simulink model "DDS_LUT_Stream_Ex1"  (R2024a)
settings: Solver=VariableStepAuto  StartTime=0.0  StopTime=0.001  RelTol=1e-3
undefined symbols (not defined in the file): i, None, S, vsva1596, xcvc1502
libraries: aieUtilities x2, hdlUtilities x1, aieDSP x1, dspsigops x1, vmcUtilities x1
settings Model: Creator=sdegala  LastModifiedBy=robg
settings ModelReferenceCC: EnableRefExpFcnMdlSchedulingChecks=on
settings RTWCC: GPUComputeCapability=3.5
settings ConfigComp: CovBoundaryAbsTol=1.0e-5

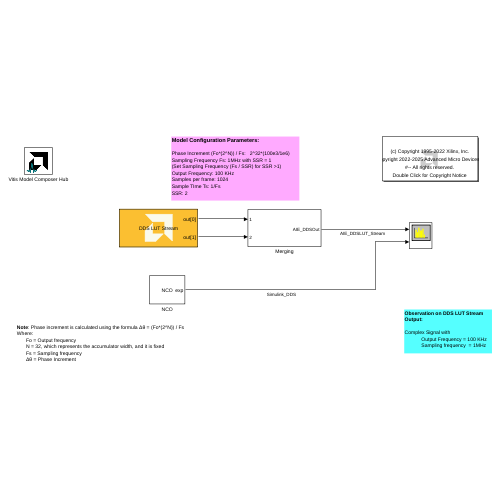
[thumbnail: Simulink's stored preview of the top-level diagram]
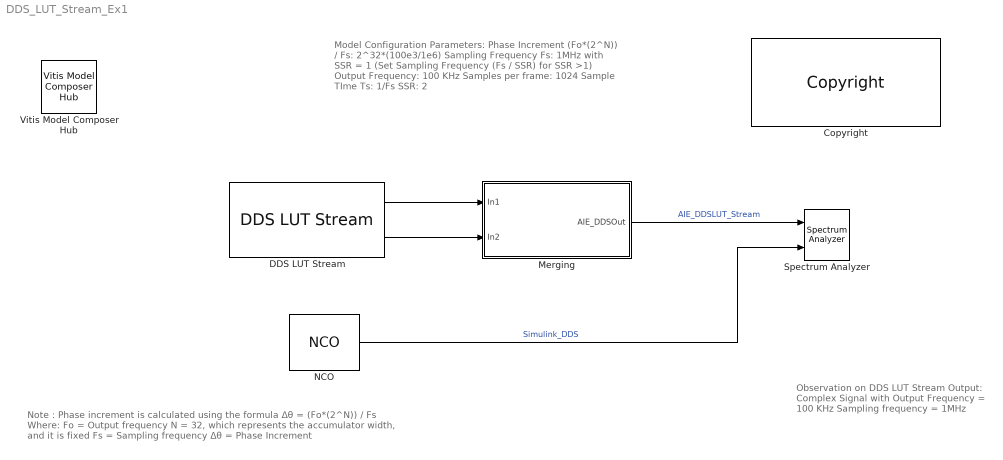
== system DDS_LUT_Stream_Ex1 ==
  note: Note : Phase increment is calculated using the formula Δθ = (Fo*(2^N)) / Fs
      | Where:
      | Fo = Output frequency
      | N = 32, which represents the accumulator width, and it is fixed
      | Fs = Sampling frequency
      | Δθ = Phase Increment
  note: Model Configuration Parameters:
      |
      | Phase Increment (Fo*(2^N)) / Fs: 2^32*(100e3/1e6)
      | Sampling Frequency Fs: 1MHz with SSR = 1
      | (Set Sampling Frequency (Fs / SSR) for SSR >1)
      | Output Frequency: 100 KHz
      | Samples per frame: 1024
      | Sample TIme Ts: 1/Fs
      | SSR: 2
  note: Observation on DDS LUT Stream Output:
      |
      | Complex Signal with
      | Output Frequency = 100 KHz
      | Sampling frequency = 1MHz
  Copyright : hdlUtilities/Copyright  copyrighttext="(c) Copyright 1995-2022 Xilinx, Inc. <br>(c) Copyright 2022-2025 Advanced Micro Devices, Inc. All rights reserved.<br><br>This document  contains proprietary, confidential information that may be used, copied and/or disclosed only as authorized by a valid licensing agreement with Advanced Micro Devices, Inc. This copyright notice must be retained on all authorized copies.<br><br> This code is provided \"as is\". Advanced Micro Devices, Inc. makes, and the end user receives, no warranties or conditions, express, implied, statutory or otherwise, and Advanced Micro Devices, Inc. specifically disclaims any implied warranties of merchantability, <br>non-infringement, or fitness for a particular purpose."  block_type=copyright
  DDS LUT Stream : aieDSP/DDS LUT Stream  AIE_VARIANT=1  data_type=cfloat  sfdr=80  vmc_ssr_inherit=off  vmc_outputcolumn=1  ssr=2  output_window_size=1024  initial_phase_offset=0  USE_PHASE_RELOAD=off  PHASE_RELOAD_API=off  phase_increment=4.2950e+08  phase_increment_reload=off  rnd_mode=Floor  sat_mode=0-None  vmc_sample_time=1/(1e6/2)  TP_API=1  MIXER_MODE=0  blockJsonConstraints=[]  blockJsonConstraintsInternal=[]  spec=vmc_stream_dds_lut.json  SerializedMaskParamNames=[]  SerializedMaskParamValues=[]  SerializedMaskParamVisibilities=[]  block_type=DDS LUT Stream  SerializedMaskParamDataypes=uint|typename|uint|uint|uint|uint|uint|uint|uint|uint|uint|uint|uint|uint|double|uint|uint  SerializedMaskParamEnumStrArr=0|0|0|0|0|0|0|0|0|0|0|0|Floor,Ceiling,Round to positive infinity,Round to negative infinity,Round symmetrical to infinity,Round symmetrical to zero,Round convergent to even,Round convergent to odd|0-None,1-Asymmetric,3-Symmetric|0|0|0  SerializedMaskParamEnumValArr=0|0|0|0|0|0|0|0|0|0|0|0|0,1,2,3,4,5,6,7|0,1,3|0|0|0  SerializedMaskParamVectorArr=0|0|0|0|0|0|0|0|0|0|0|0|0|0|0|0|0  SerializedMaskParamKeys=AIE_VARIANT|TT_DATA|TP_SFDR|vmc_ssr_inherit|vmc_outputcolumn|TP_SSR|TP_INPUT_WINDOW_VSIZE|initialPhaseOffset|TP_USE_PHASE_RELOAD|TP_PHASE_RELOAD_API|phaseInc|TP_USE_PHASE_INC_RELOAD|TP_RND|TP_SAT|vmc_sample_time|TP_API|TP_MIXER_MODE
  Merging : Subsystem
  NCO : dspsigops/NCO  AccIncSrc=Specify via dialog  AccInc=4.2950e+08  PhaseOffsetSrc=Specify via dialog  PhaseOffset=0  AccumWL=32  HasDither=off  DitherWL=4  PNgeneratorLength=19  HasPhaseQuantizer=on  TableDepth=16  HasOutputPhaseError=off  Formula=Complex exponential  DataType=single  OutputWL=16  OutputFL=15  CompMethod=Table lookup (no interpolation)  SampleTime=1/1e6  SamplesPerFrame=1024  OutputFrames=off
  Spectrum Analyzer : SpectrumAnalyzer  NumInputPorts=2  WindowPosition=[1.000000,1.000000,1280.000000,744.000000,]  Visible=on  ScopeFrameLocation=window  Span=1000000  StartFrequency=-500000  StopFrequency=500000  YLimits=[-37.91126897,34.84558591]  ShowLegend=on
  Vitis Model Composer Hub : vmcUtilities/Vitis Model Composer Hub  Tag=genX  CodeGeneration=off  StartColumn=1  NumberOfColumns=1  TargetDirectory=./code  exportDesign=off  analyzeDesign=off  validateDesignOnHw=off  ExportType=AI Engines  IpVendor=xilinx.com  IpLibrary=hls  IpVersion=1.0  IpHWLanguage=Verilog  AieCompilerOptions={}  AieSimulatorOptions={}  CreateTestbench=off  TestbenchStackSize=10  RunRtlSim=off  RunCSim=off  RunAieSim=off  AieSimTimeout=50000  RunAieSimProfiling=off  LaunchVitisAnalyzer=off  PlotOutput=off  RunX86Sim=off  X86SimTimeout=10  GenHwImage=off  GenLibadfXo=off  GenHwValidationCode=off  PlatformType=Not Specified  HwSystemType=Baremetal  HwValidationTarget=hw  ProjDevice=xcvc1502-vsva1596-2HP-i-S  ProjDevicePart=xcvc1502-vsva1596-2HP-i-S  AIEType=AIE  SamplePeriod=-1  ClockFrequency=200  DataPathParallelism=1  xilinxfamily=versalaicore  part=xcvc1502  speed=-2HP-i-S  package=vsva1596  directory=./netlist  testbench=off  incr_netlist=off  synthesis_tool=Vivado  clock_wrapper=Clock Enables  dbl_ovrd=According to Block Masks  dcm_input_clock_period=10  sysclk_period=10  simulink_period=1  eval_field=0  LogFileName=''  NThreads=4
  wires:
  NCO/1 -> Spectrum Analyzer/2  "Simulink_DDS"
  DDS LUT Stream/1 -> Merging/1(In1)
  DDS LUT Stream/2 -> Merging/2(In2)
  Merging/1(AIE_DDSOut) -> Spectrum Analyzer/1  "AIE_DDSLUT_Stream"

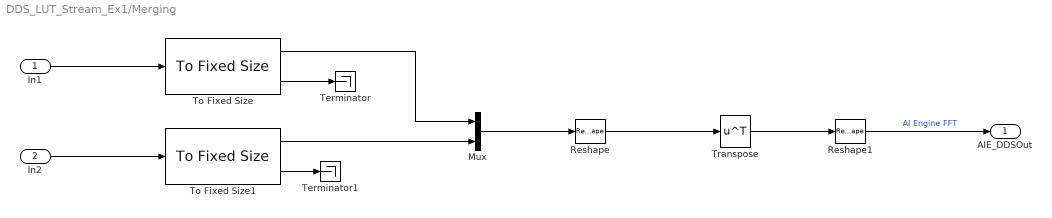
== system DDS_LUT_Stream_Ex1/Merging ==
  In1 : Inport
  In2 : Inport  Port=2
  Mux : Mux  Inputs=2
  Reshape : Reshape  OutputDimensionality=Customize  OutputDimensions=[512, 2]
  Reshape1 : Reshape  OutputDimensions=[1, 10]
  Terminator : Terminator
  Terminator1 : Terminator
  To Fixed Size : aieUtilities/To Fixed Size  Mode=Produce a valid output signal  OutputSize=Inherit: Same as input  CopyMethod=Buffer samples to form output  HasStatusOutput=on
  To Fixed Size1 : aieUtilities/To Fixed Size  Mode=Produce a valid output signal  OutputSize=Inherit: Same as input  CopyMethod=Buffer samples to form output  HasStatusOutput=on
  Transpose : Math  Operator=transpose
  AIE_DDSOut : Outport
  wires:
  Reshape/1 -> Transpose/1
  To Fixed Size1/2 -> Terminator1/1
  To Fixed Size1/1 -> Mux/2
  In2/1 -> To Fixed Size1/1
  To Fixed Size/2 -> Terminator/1
  Transpose/1 -> Reshape1/1
  To Fixed Size/1 -> Mux/1
  Mux/1 -> Reshape/1
  Reshape1/1 -> AIE_DDSOut/1  "AI Engine FFT"
  In1/1 -> To Fixed Size/1
